simulink model "MPC_mobile_base_KIN_IPOPT_ROS"  (R2018b)
settings: Solver=ode4  StartTime=0.0  StopTime=inf  FixedStep=Tsample  RelTol=1e-3
values from neighbouring files (symbols this model uses):
  N = length(q)    [FK.m]    (also in FK_generation.m = size(DHTABLE,1); init_prova_vera1.mat = 10; init_prova_vera3.mat = 10; jacobian_MM.m)
  T = cell(N+1,1)    [FK.m]    (also in init_prova_vera1.mat = 0.5; init_prova_vera3.mat = 0.5; jacobian_MM.m; matlabultimo.mat = 0.5)
  xd = [0 0 0 0 0 0 0 0 0 0.0238792670666 0.415141969475 1.22261425872 ... (1458 elements, 18x81)]    [init_prova_vera1.mat]    (also in init_prova_vera3.mat; liveplot.m = evalin('base','xd'); matlabultimo.mat = [0 0 0 0 0 0 0 0 0 -0.528285242967 -0.106449885857 1.3372295; prova_vera1.mat)
undefined symbols (not defined in the file or in its folder): Angular, Linear
libraries: robotlib x3, simulink x2, sharedtransform x1, templibrary x1
settings Model: Creator=francesco  LastModifiedBy=francesco

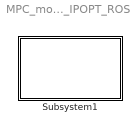
== system MPC_mobile_base_KIN_IPOPT_ROS ==
  Subsystem1 : Subsystem  InitFcn=|
      | clearvars -EXCEPT  xd N T Tsample tt
      | 
      | import casadi.*
      | 
      | 
      | %%%%%%%%%%%% SETTINGS %%%%%%%%%%%%%%%%%%%%%
      | 
      | fs = 1/T; % Sampling frequency [hz]
      | m  = 2;
      | T_horizon=(0:N-1)*T;
      | 
      | Ak= diag([10    10    50]);
      | 
      | Vpmax=inf;  %  [m/s^2]
      | Wpmax=3; %  [rad/s^2]
      | 
      | Vpmax=Vpmax*T;
      | Wpmax=Wpmax*T;
      | %%%%%%%%%%%% MODELING %%%%%%%%%%%%%%%%%%%%%
      | x  = MX.sym('x',3);
      | Xd  = MX.sym('Xd',3,N);
      | t  = MX.sym('t');
      | x0 = MX.sym('x0',3);
      | U0  = MX.sym('U0',2,1);
      | 
      | p = MX.sym('p',8);
      | 
      | % xdot = [(p(1)*t^2+p(2)*t+p(3))*cos(x(3)); ...
      | %         (p(1)*t^2+p(2)*t+p(3))*sin(x(3)); ...
      | %         (p(4)*t^3+p(5)*t^2+p(6)*t+p(7))         ];
      | 
      | xdot = [(p(1)*t^3+p(2)*t^2+p(3)*t+p(4))*cos(x(3)); ...
      |         (p(1)*t^3+p(2)*t^2+p(3)*t+p(4))*sin(x(3)); ...
      |         (p(5)*t^3+p(6)*t^2+p(7)*t+p(8))         ];
      | 
      | % Form an ode function
      | ode = Function('ode',{x,p,t},{xdot});
      | 
      | %%%%%%%%%%%% Creating a simulator %%%%%%%%%%
      | N_steps_per_sample = 2;
      | dt = 1/fs/N_steps_per_sample;
      | 
      | % Build an integrator for this system: Runge Kutta 4 integrator
      | k1 = ode(x,p,t);
      | k2 = ode(x+dt/2.0*k1,p,t+dt/2.0);
      | k3 = ode(x+dt/2.0*k2,p,t+dt/2.0);
      | k4 = ode(x+dt*k3,p,t+dt/2.0);
      | 
      | xstep = x+dt/6.0*(k1+2*k2+2*k3+k4);
      | 
      | % Create a function that simulates one step propagation in a sample
      | one_step = Function('one_step',{x, p, t},{xstep});
      | 
      | X = x;
      | for i=1:N_steps_per_sample
      |     X = one_step(X, p, t);
      | end
      | 
      | % Create a function that simulates all step propagation on a sample
      | one_sample = Function('one_sample',{x, p, t}, {X});
      | 
      | % speedup trick: expand into scalar operations
      | one_sample = one_sample.expand();
      | 
      | 
      | %%%%%%%%%%%% Simulating the system %%%%%%%%%%
      | 
      | all_samples = one_sample.mapaccum('all_samples', N);
      | 
      | %%%%%%%%%%%% Identifying the simulated system: single shooting strategy %%%%%%%%%%
      | 
      | % Note, it is in general a good idea to scale your decision variables such
      | % that they are in the order of ~0.1..100
      | X_forecast = [all_samples(x0, repmat(p,1,N),T_horizon)];
      | 
      | usym = [p(1)*t^3+p(2)*t^2+p(3)*t+p(4); ...
      |         p(5)*t^3+p(6)*t^2+p(7)*t+p(8)];
      |     
      | Usym=Function('Usym',{p,t},{usym});
      | 
      | J=0;
      | g={};
      | lbg=[];
      | ubg=[];
      | 
      | for i=1:N
      | 
      | ex=(X_forecast(1,i)-Xd(1,i));
      | ey=(X_forecast(2,i)-Xd(2,i));
      | eth=(X_forecast(3,i)-Xd(3,i));
      |     
      | J = J + ((i/N)^m)*abs([ex ey eth]*Ak*[ex ey eth].');
      | 
      | if i==1
      |     
      | g = {g{:}, Usym(p,T_horizon(i))-U0 };
      | 
      | else
      |     
      | g = {g{:}, Usym(p,T_horizon(i))-Usym(p,T_horizon(i-1)) };
      | 
      | end
      | 
      | lbg = [lbg; [-Vpmax -Wpmax].'];
      | ubg = [ubg; [ Vpmax  Wpmax].'];
      | 
      | end
      | 
      | Gfunction=Function('Gfunction',{p,U0}, {vertcat(g{:})});
      | 
      | Costfunction=Function('Costfunction',{Xd,p,x0}, {J});
      | 
      | % nlp = struct('x', p, 'f', Costfunction(xd_val,p));%, 'g', G);
      | % solver = nlpsol('solver','ipopt', nlp);
      | % 
      | % 
      | % sol = solver('x0',p0);

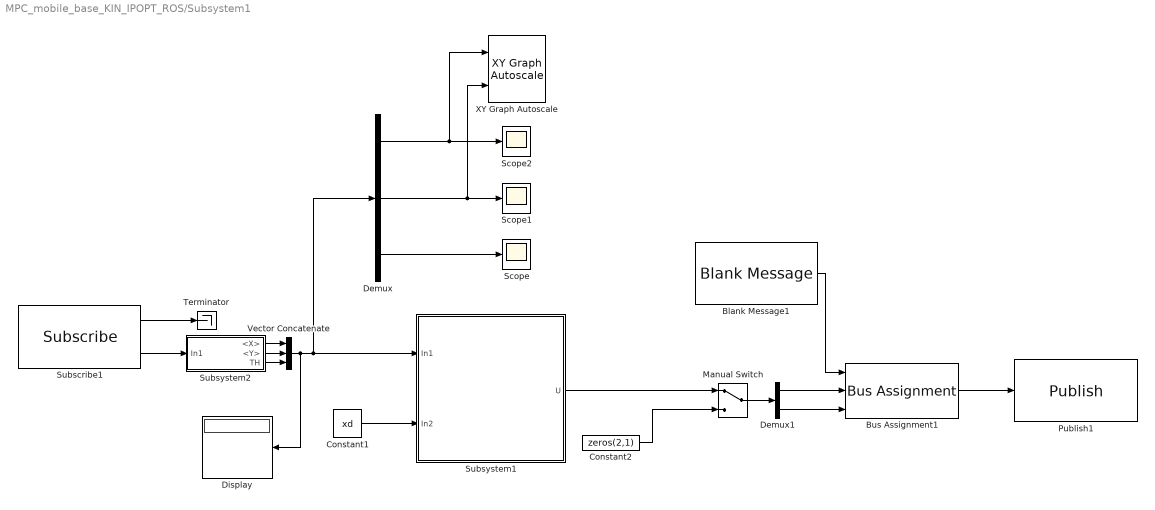
== system MPC_mobile_base_KIN_IPOPT_ROS/Subsystem1 ==
  Blank Message1 : robotlib/Blank Message  messageClass=Message  entityType=geometry_msgs/Twist  messageType=geometry_msgs/Twist  SampleTime=T
      settings: SourceProductBaseCode=RO
  Bus Assignment1 : BusAssignment  AssignedSignals=Linear.X,Angular.Z
  Constant1 : Constant  Value=xd
  Constant2 : Constant  Value=zeros(2,1)
  Demux : Demux  Outputs=3
  Demux1 : Demux  Outputs=2
  Display : Display
  Manual Switch : ManualSwitch
  Publish1 : robotlib/Publish  topicSource=Select from ROS network  topic=/cmd_vel  messageType=geometry_msgs/Twist  messageQueueLength=1
      settings: SourceProductBaseCode=RO
  Scope : Scope
  Scope1 : Scope
  Scope2 : Scope
  Subscribe1 : robotlib/Subscribe  topicSource=Select from ROS network  topic=/odom  messageType=nav_msgs/Odometry  sampleTime=T  messageQueueLength=1
      settings: SourceProductBaseCode=RO
  Subsystem1 : Subsystem
  Subsystem2 : Subsystem
  Terminator : Terminator
  Vector Concatenate : Concatenate  NumInputs=3
  XY Graph Autoscale : templibrary/XY Graph  Autoscale  xmin=-1  xmax=1  ymin=-1  ymax=1  st=-1
  wires:
  Demux/1 -> Scope2/1, XY Graph Autoscale/1
  Demux/3 -> Scope/1
  Demux/2 -> Scope1/1, XY Graph Autoscale/2
  Constant1/1 -> Subsystem1/2(In2)
  Subscribe1/2 -> Subsystem2/1(In1)
  Subsystem2/1(<X>) -> Vector Concatenate/1
  Subsystem2/2(<Y>) -> Vector Concatenate/2
  Vector Concatenate/1 -> Demux/1, Subsystem1/1(In1), Display/1
  Subsystem2/3(TH) -> Vector Concatenate/3
  Subscribe1/1 -> Terminator/1
  Constant2/1 -> Manual Switch/2
  Manual Switch/1 -> Demux1/1
  Subsystem1/1(U) -> Manual Switch/1
  Bus Assignment1/1 -> Publish1/1
  Blank Message1/1 -> Bus Assignment1/1
  Demux1/2 -> Bus Assignment1/3
  Demux1/1 -> Bus Assignment1/2

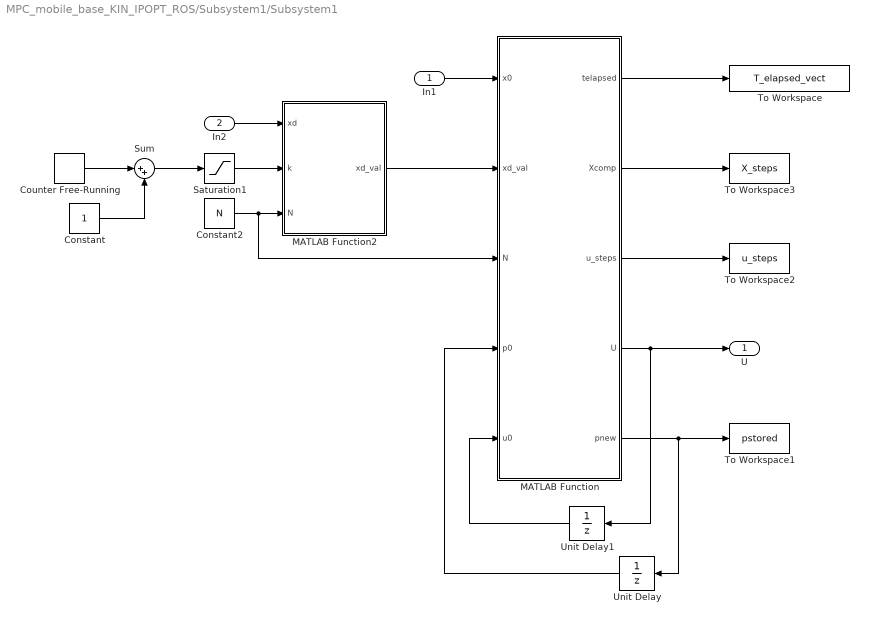
== system MPC_mobile_base_KIN_IPOPT_ROS/Subsystem1/Subsystem1 ==
  In1 : Inport
  In2 : Inport  Port=2
  Constant : Constant
  Constant2 : Constant  Value=N
  Counter Free-Running : simulink/Sources/Counter Free-Running  NumBits=12  tsamp=T
  MATLAB Function : MATLAB Function  TreatAsAtomicUnit=on
  MATLAB Function2 : MATLAB Function  TreatAsAtomicUnit=on
  Saturation1 : Saturate  UpperLimit=size(xd,2)
  Sum : Sum  Inputs=|++
  To Workspace : ToWorkspace  VariableName=T_elapsed_vect  SampleTime=T
  To Workspace1 : ToWorkspace  VariableName=pstored  SampleTime=-1
  To Workspace2 : ToWorkspace  VariableName=u_steps  SaveFormat=Structure  SampleTime=-1
  To Workspace3 : ToWorkspace  VariableName=X_steps  SaveFormat=Structure  SampleTime=-1
  Unit Delay : UnitDelay  InitialCondition=[0 0 0 0.1 0 0 0 0].'  SampleTime=T
  Unit Delay1 : UnitDelay  InitialCondition=[0 0].'  SampleTime=T
  U : Outport
  wires:
  Counter Free-Running/1 -> Sum/1
  MATLAB Function/5(pnew) -> To Workspace1/1, Unit Delay/1
  Sum/1 -> Saturation1/1
  Constant/1 -> Sum/2
  In1/1 -> MATLAB Function/1(x0)
  Constant2/1 -> MATLAB Function/3(N), MATLAB Function2/3(N)
  In2/1 -> MATLAB Function2/1(xd)
  MATLAB Function/4(U) -> Unit Delay1/1, U/1
  Unit Delay/1 -> MATLAB Function/4(p0)
  Saturation1/1 -> MATLAB Function2/2(k)
  MATLAB Function2/1(xd_val) -> MATLAB Function/2(xd_val)
  MATLAB Function/1(telapsed) -> To Workspace/1
  Unit Delay1/1 -> MATLAB Function/5(u0)
  MATLAB Function/3(u_steps) -> To Workspace2/1
  MATLAB Function/2(Xcomp) -> To Workspace3/1

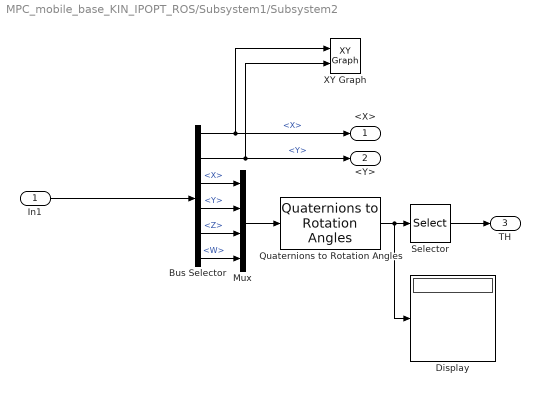
== system MPC_mobile_base_KIN_IPOPT_ROS/Subsystem1/Subsystem2 ==
  In1 : Inport
  Bus Selector : BusSelector  OutputSignals=Pose.Pose.Position.X,Pose.Pose.Position.Y,Pose.Pose.Orientation.X,Pose.Pose.Orientation.Y,Pose.Pose.Orientation.Z,Pose.Pose.Orientation.W
  Display : Display
  Mux : Mux
  Quaternions to Rotation Angles : sharedtransform/Quaternions to Rotation Angles  rotationOrder=ZYX  aMode=aMode
      settings: SourceProductBaseCode=AE
  Selector : Selector  InputPortWidth=3  IndexOptions=Index vector (dialog)  Indices=3  OutputSizes=1
  XY Graph : simulink/Sinks/XY Graph  xmin=-1  xmax=10  ymin=-1  ymax=4  st=-1
  <X> : Outport
  <Y> : Outport  Port=2
  TH : Outport  Port=3
  wires:
  Bus Selector/1 -> XY Graph/1, <X>/1  "<X>"
  In1/1 -> Bus Selector/1
  Bus Selector/2 -> XY Graph/2, <Y>/1  "<Y>"
  Bus Selector/6 -> Mux/4  "<W>"
  Bus Selector/5 -> Mux/3  "<Z>"
  Bus Selector/4 -> Mux/2  "<Y>"
  Bus Selector/3 -> Mux/1  "<X>"
  Mux/1 -> Quaternions to Rotation Angles/1
  Quaternions to Rotation Angles/1 -> Display/1, Selector/1
  Selector/1 -> TH/1

== matlab function MPC_mobile_base_KIN_IPOPT_ROS/Subsystem1/Subsystem1/MATLAB Function ==
  settings: updateMethod=DISCRETE  sampleTime=T
  data: telapsed output; Xcomp output size=[3,N+1]; u_steps output size=[3,N]; U output; x0 input; pnew output; xd_val input; N input; p0 input; u0 input
function [telapsed,Xcomp,u_steps,U,pnew] = fnc(x0,xd_val,N,p0,u0)

telapsed=0;
u_steps=zeros(2,N);

coder.extrinsic('solver_NLP');

pnew=zeros(8,1);
U=zeros(2,1);
Xcomp=zeros(3,N);

[pnew, U, u_steps, Xcomp, telapsed] = solver_NLP(xd_val,p0,x0,u0);


end

== matlab function MPC_mobile_base_KIN_IPOPT_ROS/Subsystem1/Subsystem1/MATLAB Function2 ==
  settings: updateMethod=DISCRETE  sampleTime=T
  data: xd input; k input; N input; xd_val output size=[3,N]
function xd_val = fcn(xd,k,N)

xd_val=zeros(3,N);

if size(xd,2)-k>N-1
h=xd(:,k+1:k+N);
      
else
h=[xd(:,k+1:end) xd(:,end)*ones(1,N-(size(xd,2)-k))];

end
xd_val = h;

end
